simulink model "motor_velocity_2dof"  (R2014b)
settings: Solver=VariableStepAuto  StartTime=0.0  StopTime=simtime  RelTol=1e-3
values from neighbouring files (symbols this model uses):
  enable_karnop = 0    [discrete_velocity.m]    (also in ex1.m = 1; motor_parameters.mat = 1; pcontrol.m; pcontrol_position.m)
  enable_sin = 0    [discrete_velocity.m]    (also in ex1.m = 1; motor_parameters.mat; pcontrol.m = 1; pcontrol_position.m = 1)
  F_c = 1e-3    (= 0.001)    [ex1.m]    (also in motor_parameters.mat; position_ctrl.m; velocity_ctrl.m)
  J = J1+J2    (= 3.6e-05)    [ex1.m]    (also in lec_example.m = 0.1; position_ctrl.m = motor.J; velocity_ctrl.m)
  motor = motor_pars    [ex1.m]    (also in position_ctrl.m; velocity_ctrl.m)
  n = 5    [ex1.m]    (also in motor_parameters.mat; position_ctrl.m; velocity_ctrl.m)
  R = 1    [pcontrol.m]    (also in pcontrol_position.m; pdcontroller_position.m = [1 r0]; picontroller.m = [1 0]; picontroller_position.m = [1 r0])
  S = P    (= 8)    [pcontrol.m]    (also in pcontrol_position.m = 4; pdcontroller_position.m = [s1 s0]; picontroller.m = [P I]; picontroller_position.m = [s1 s0])
  sim_sin_amp = 200    [ex1.m]    (also in motor_parameters.mat = 1; pcontrol.m = 10; pcontrol_position.m = 10; pdcontroller_position.m = 10)
  sim_sin_freq = 10    [ex1.m]    (also in motor_parameters.mat = 1; pcontrol.m = 1; pcontrol_position.m = 1; pdcontroller_position.m = 1)
  sim_v = Vmax    (= 24)    [ex1.m]    (also in motor_parameters.mat; pcontrol.m = 1; pcontrol_position.m = 1; pdcontroller_position.m = 1)
  T = P    (= 8)    [pcontrol.m]    (also in pcontrol_position.m = 4; pdcontroller_position.m = S; picontroller.m = t0*[1 omega2]; picontroller_position.m = S)
libraries: simulink x2
settings Model: Creator=Gabriel  LastModifiedBy=gabras
settings DataIOCC: SaveFormat=Dataset
settings OptimizationCC: UseDivisionForNetSlopeComputation=off  SimCompilerOptimization=off
settings DebuggingCC: SolverPrmCheckMsg=none  FrameProcessingCompatibilityMsg=error  AllowSymbolicDim=off
settings HardwareCC: ProdBitPerPointer=64  ProdLargestAtomicFloat=Float  ProdIntDivRoundTo=Zero  ProdEndianess=LittleEndian  ProdWordSize=64  ProdHWDeviceType=Intel->x86-64 (Windows64)
settings RTWCC: RTWCompilerOptimization=off
settings GRTTargetCC: GeneratePreprocessorConditionals=Use local settings
settings ConfigComp: CovMetricSettings=dw  CovHtmlReporting=on  CovSaveCumulativeToWorkspaceVar=on  CovSaveSingleToWorkspaceVar=on  CovExternalEMLEnable=off

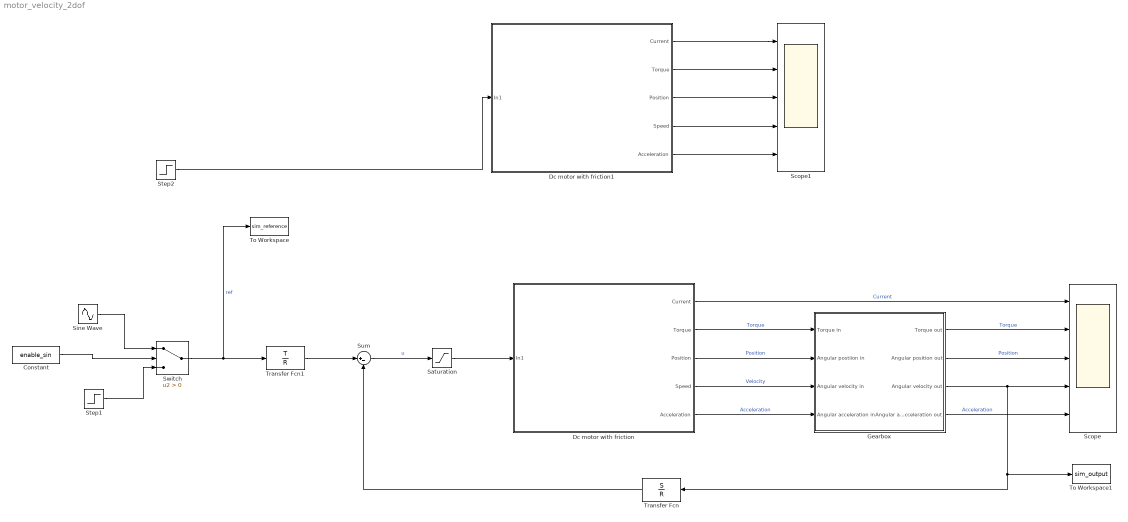
== system motor_velocity_2dof ==
  Constant : Constant  Value=enable_sin
  Dc motor with friction : Subsystem
      mask Display:
      | image('dcmotor.jpg')
      | port_label('input', 1, 'Voltage')
      | port_label('output', 1, 'Current')
      | port_label('output', 2, 'Torque')
      | port_label('output', 3, 'Position')
      | port_label('output', 4, 'Velocity')
      | port_label('output', 5, 'Acceleration')
  Dc motor with friction1 : Subsystem
      mask Display:
      | image('dcmotor.jpg')
      | port_label('input', 1, 'Voltage')
      | port_label('output', 1, 'Current')
      | port_label('output', 2, 'Torque')
      | port_label('output', 3, 'Position')
      | port_label('output', 4, 'Velocity')
      | port_label('output', 5, 'Acceleration')
  Gearbox : Subsystem
  Saturation : Saturate  UpperLimit=24  LowerLimit=-24
  Scope : Scope  NumInputPorts=5
      settings: YMin=-0.7198~-0.25085~-1.49914~-4.86523~-4731.79  YMax=1.13271~0.39475~13.4923~43.7871~7102.06
  Scope1 : Scope  NumInputPorts=5
      settings: YMin=-0.7198~-0.25085~-1.49914~-4.86523~-4731.79  YMax=1.13271~0.39475~13.4923~43.7871~7102.06
  Sine Wave : Sin  Amplitude=sim_sin_amp  Frequency=sim_sin_freq  SampleTime=0
  Step1 : Step  Time=0  After=sim_v  SampleTime=0
  Step2 : Step  Time=0  SampleTime=0
  Sum : Sum  Inputs=|+-
  Switch : Switch  Criteria=u2 > Threshold
  To Workspace : ToWorkspace  VariableName=sim_reference  SaveFormat=Timeseries  SampleTime=-1
  To Workspace1 : ToWorkspace  VariableName=sim_output  SaveFormat=Timeseries  SampleTime=-1
  Transfer Fcn : TransferFcn  Numerator=S  Denominator=R
  Transfer Fcn1 : TransferFcn  Numerator=T  Denominator=R
  wires:
  Step1/1 -> Switch/3
  Sine Wave/1 -> Switch/1
  Constant/1 -> Switch/2
  Switch/1 -> Transfer Fcn1/1, To Workspace/1  "ref"
  Dc motor with friction/4(Speed) -> Gearbox/3(Angular velocity in)  "Velocity"
  Dc motor with friction/2(Torque) -> Gearbox/1(Torque in)  "Torque"
  Dc motor with friction/1(Current) -> Scope/1  "Current"
  Dc motor with friction/5(Acceleration) -> Gearbox/4(Angular acceleration in)  "Acceleration"
  Dc motor with friction/3(Position) -> Gearbox/2(Angular postiion in)  "Position"
  Gearbox/1(Torque out) -> Scope/2  "Torque"
  Gearbox/2(Angular position out) -> Scope/3  "Position"
  Gearbox/3(Angular velocity out) -> To Workspace1/1, Transfer Fcn/1, Scope/4
  Gearbox/4(Angular acceleration out) -> Scope/5  "Acceleration"
  Transfer Fcn/1 -> Sum/2
  Transfer Fcn1/1 -> Sum/1
  Sum/1 -> Saturation/1  "u"
  Dc motor with friction1/1(Current) -> Scope1/1
  Dc motor with friction1/2(Torque) -> Scope1/2
  Dc motor with friction1/3(Position) -> Scope1/3
  Dc motor with friction1/4(Speed) -> Scope1/4
  Dc motor with friction1/5(Acceleration) -> Scope1/5
  Step2/1 -> Dc motor with friction1/1(In1)
  Saturation/1 -> Dc motor with friction/1(In1)

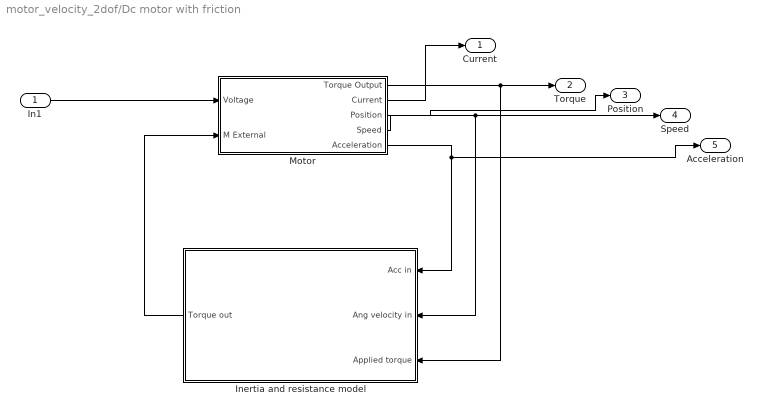
== system motor_velocity_2dof/Dc motor with friction ==
  In1 : Inport
  "Inertia and resistance model " : Subsystem
  Motor : Subsystem
  Current : Outport
  Torque : Outport  Port=2
  Position : Outport  Port=3
  Speed : Outport  Port=4
  Acceleration : Outport  Port=5
  wires:
  Motor/4(Speed) -> Speed/1, "Inertia and resistance model "/2(Ang velocity in)
  Motor/3(Position) -> Position/1
  Motor/2(Current) -> Current/1
  "Inertia and resistance model "/1(Torque out) -> Motor/2("M External ")
  Motor/1(Torque Output) -> Torque/1, "Inertia and resistance model "/3(Applied torque)
  In1/1 -> Motor/1(Voltage)
  Motor/5(Acceleration) -> "Inertia and resistance model "/1(Acc in), Acceleration/1

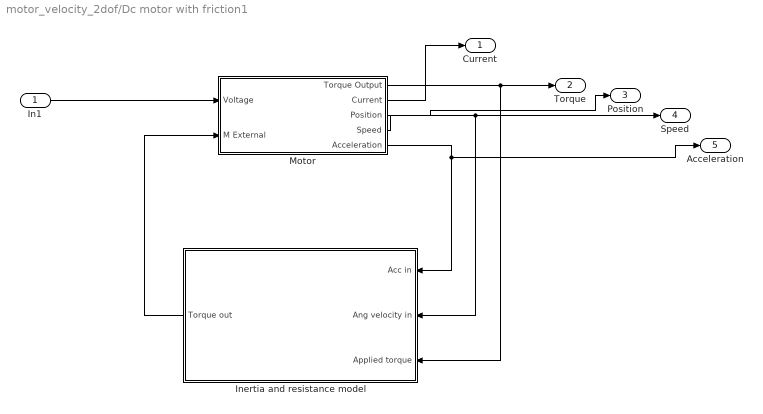
== system motor_velocity_2dof/Dc motor with friction1 ==
  In1 : Inport
  "Inertia and resistance model " : Subsystem
  Motor : Subsystem
  Current : Outport
  Torque : Outport  Port=2
  Position : Outport  Port=3
  Speed : Outport  Port=4
  Acceleration : Outport  Port=5
  wires:
  Motor/5(Acceleration) -> Acceleration/1, "Inertia and resistance model "/1(Acc in)
  In1/1 -> Motor/1(Voltage)
  Motor/1(Torque Output) -> "Inertia and resistance model "/3(Applied torque), Torque/1
  "Inertia and resistance model "/1(Torque out) -> Motor/2("M External ")
  Motor/2(Current) -> Current/1
  Motor/3(Position) -> Position/1
  Motor/4(Speed) -> "Inertia and resistance model "/2(Ang velocity in), Speed/1

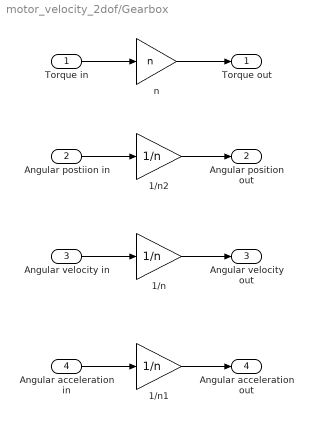
== system motor_velocity_2dof/Gearbox ==
  Torque in : Inport
  Angular postiion in : Inport  Port=2
  Angular velocity in : Inport  Port=3
  Angular acceleration in : Inport  Port=4
  1/n : Gain  Gain=1/n
  1/n1 : Gain  Gain=1/n
  1/n2 : Gain  Gain=1/n
  n : Gain  Gain=n
  Torque out : Outport
  Angular position out : Outport  Port=2
  Angular velocity out : Outport  Port=3
  Angular acceleration out : Outport  Port=4
  wires:
  1/n/1 -> Angular velocity out/1
  Angular velocity in/1 -> 1/n/1
  n/1 -> Torque out/1
  Torque in/1 -> n/1
  1/n1/1 -> Angular acceleration out/1
  Angular acceleration in/1 -> 1/n1/1
  1/n2/1 -> Angular position out/1
  Angular postiion in/1 -> 1/n2/1

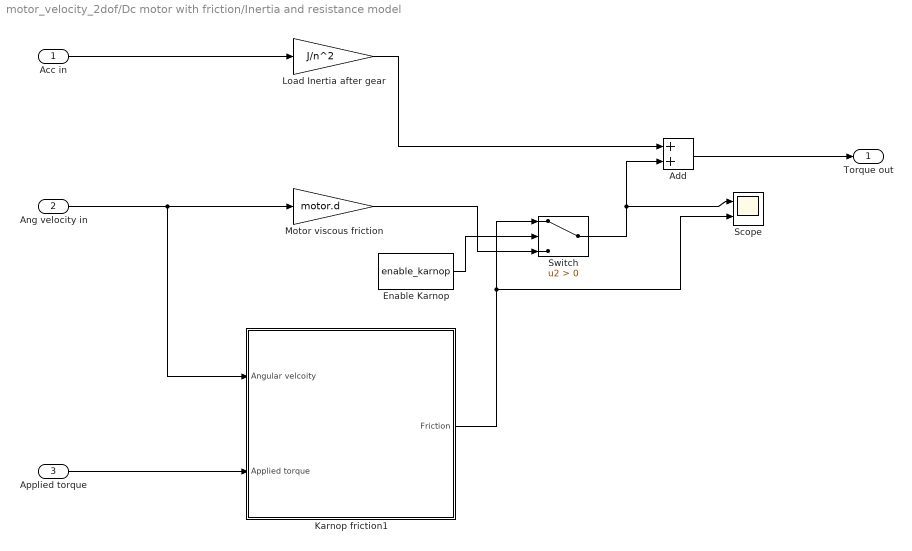
== system motor_velocity_2dof/Dc motor with friction/Inertia and resistance model  ==
  Acc in : Inport
  Ang velocity in : Inport  Port=2
  Applied torque : Inport  Port=3
  Add : Sum
  Enable Karnop : Constant  Value=enable_karnop
  Karnop friction1 : Subsystem
  Load Inertia after gear : Gain  Gain=J/n^2
  Motor viscous friction : Gain  Gain=motor.d
  Scope : Scope  NumInputPorts=2
      settings: YMin=-0.00177~-0.00177  YMax=0.00177~0.00177
  Switch : Switch  Criteria=u2 > Threshold
  Torque out : Outport
  wires:
  Acc in/1 -> Load Inertia after gear/1
  Add/1 -> Torque out/1
  Load Inertia after gear/1 -> Add/1
  Ang velocity in/1 -> Karnop friction1/1(Angular velcoity), Motor viscous friction/1
  Motor viscous friction/1 -> Switch/3
  Karnop friction1/1(Friction) -> Switch/1, Scope/2
  Switch/1 -> Add/2, Scope/1
  Enable Karnop/1 -> Switch/2
  Applied torque/1 -> Karnop friction1/2("Applied torque ")

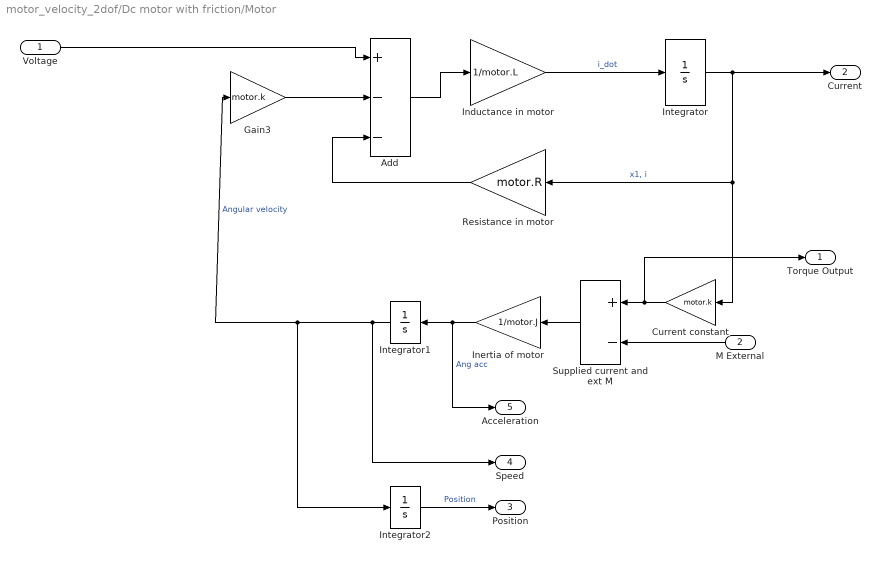
== system motor_velocity_2dof/Dc motor with friction/Motor ==
  Voltage : Inport
  "M External " : Inport  Port=2
  Add : Sum  Inputs=+--
  Current constant : Gain  Gain=motor.k
  Gain3 : Gain  Gain=motor.k
  Inductance in motor : Gain  Gain=1/motor.L
  Inertia of motor : Gain  Gain=1/motor.J
  Integrator : Integrator
  Integrator1 : Integrator
  Integrator2 : Integrator
  Resistance in motor : Gain  Gain=motor.R
  "Supplied current and ext M " : Sum  Inputs=+-
  Torque Output : Outport
  Current : Outport  Port=2
  Position : Outport  Port=3
  Speed : Outport  Port=4
  Acceleration : Outport  Port=5
  wires:
  Voltage/1 -> Add/1
  Add/1 -> Inductance in motor/1
  Inductance in motor/1 -> Integrator/1  "i_dot"
  Integrator/1 -> Current constant/1, Resistance in motor/1, Current/1  "x1, i"
  Resistance in motor/1 -> Add/3
  Gain3/1 -> Add/2
  Integrator1/1 -> Speed/1, Integrator2/1, Gain3/1  "Angular velocity"
  "Supplied current and ext M "/1 -> Inertia of motor/1
  Inertia of motor/1 -> Acceleration/1, Integrator1/1  "Ang acc"
  Current constant/1 -> Torque Output/1, "Supplied current and ext M "/1
  "M External "/1 -> "Supplied current and ext M "/2
  Integrator2/1 -> Position/1  "Position"

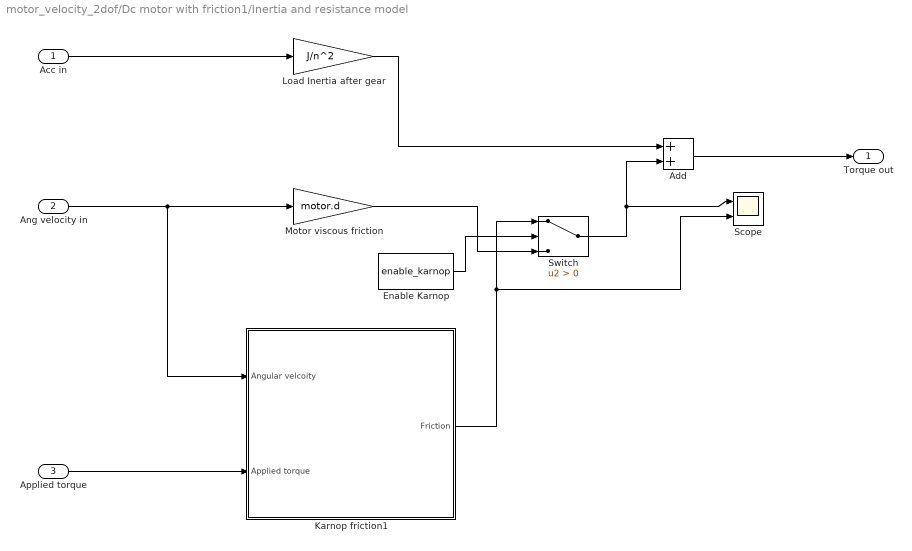
== system motor_velocity_2dof/Dc motor with friction1/Inertia and resistance model  ==
  Acc in : Inport
  Ang velocity in : Inport  Port=2
  Applied torque : Inport  Port=3
  Add : Sum
  Enable Karnop : Constant  Value=enable_karnop
  Karnop friction1 : Subsystem
  Load Inertia after gear : Gain  Gain=J/n^2
  Motor viscous friction : Gain  Gain=motor.d
  Scope : Scope  NumInputPorts=2
      settings: YMin=-0.00177~-0.00177  YMax=0.00177~0.00177
  Switch : Switch  Criteria=u2 > Threshold
  Torque out : Outport
  wires:
  Applied torque/1 -> Karnop friction1/2("Applied torque ")
  Enable Karnop/1 -> Switch/2
  Switch/1 -> Scope/1, Add/2
  Karnop friction1/1(Friction) -> Scope/2, Switch/1
  Motor viscous friction/1 -> Switch/3
  Ang velocity in/1 -> Motor viscous friction/1, Karnop friction1/1(Angular velcoity)
  Load Inertia after gear/1 -> Add/1
  Add/1 -> Torque out/1
  Acc in/1 -> Load Inertia after gear/1

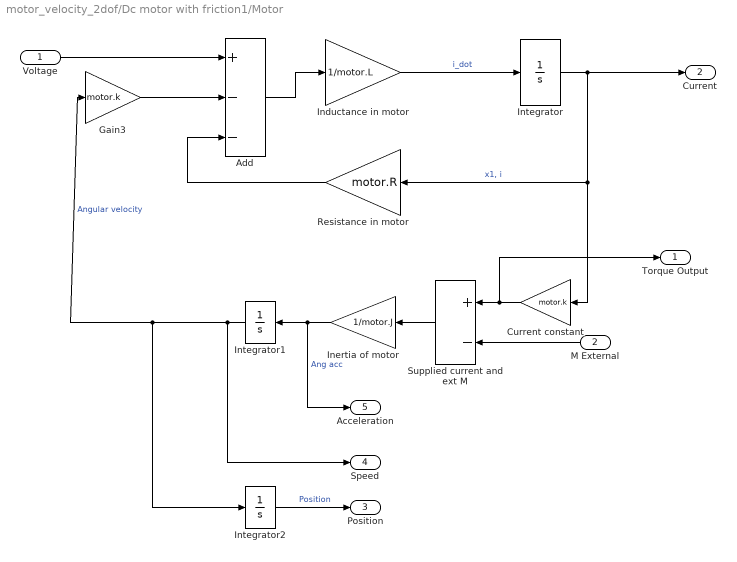
== system motor_velocity_2dof/Dc motor with friction1/Motor ==
  Voltage : Inport
  "M External " : Inport  Port=2
  Add : Sum  Inputs=+--
  Current constant : Gain  Gain=motor.k
  Gain3 : Gain  Gain=motor.k
  Inductance in motor : Gain  Gain=1/motor.L
  Inertia of motor : Gain  Gain=1/motor.J
  Integrator : Integrator
  Integrator1 : Integrator
  Integrator2 : Integrator
  Resistance in motor : Gain  Gain=motor.R
  "Supplied current and ext M " : Sum  Inputs=+-
  Torque Output : Outport
  Current : Outport  Port=2
  Position : Outport  Port=3
  Speed : Outport  Port=4
  Acceleration : Outport  Port=5
  wires:
  Integrator2/1 -> Position/1  "Position"
  "M External "/1 -> "Supplied current and ext M "/2
  Current constant/1 -> "Supplied current and ext M "/1, Torque Output/1
  Inertia of motor/1 -> Integrator1/1, Acceleration/1  "Ang acc"
  "Supplied current and ext M "/1 -> Inertia of motor/1
  Integrator1/1 -> Gain3/1, Integrator2/1, Speed/1  "Angular velocity"
  Gain3/1 -> Add/2
  Resistance in motor/1 -> Add/3
  Integrator/1 -> Current/1, Resistance in motor/1, Current constant/1  "x1, i"
  Inductance in motor/1 -> Integrator/1  "i_dot"
  Add/1 -> Inductance in motor/1
  Voltage/1 -> Add/1

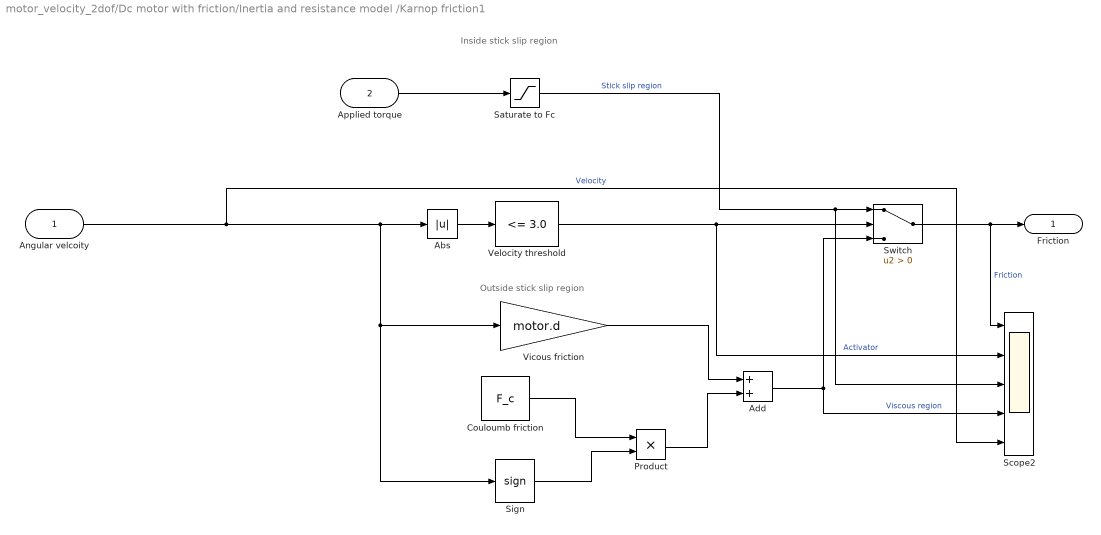
== system motor_velocity_2dof/Dc motor with friction/Inertia and resistance model /Karnop friction1 ==
  note: Inside stick slip region
  note: Outside stick slip region
  Angular velcoity : Inport
  "Applied torque " : Inport  Port=2
  Abs : Abs
  Add : Sum
  Couloumb friction : Constant  Value=F_c
  Product : Product
  Saturate to Fc : Saturate  UpperLimit=F_c  LowerLimit=-F_c
  Scope2 : Scope  NumInputPorts=5
      settings: ShowLegends=on  YMin=-0.00177~-0.125~0.0009~-0.00177~-138.1533~-0.12501~-0.12501~-0.12501  YMax=0.00177~1.125~0.0011~0.00177~138.10681~0.12501~0.12501~0.12501  SaveName=ScopeData3
  Sign : Signum
  Switch : Switch  Criteria=u2 > Threshold
  "Velocity threshold " : simulink/Logic and Bit Operations/Compare To Constant  relop=<=  const=3.0  OutDataTypeStr=boolean
  Vicous friction : Gain  Gain=motor.d
  Friction : Outport
  wires:
  Saturate to Fc/1 -> Scope2/3, Switch/1  "Stick slip region"
  Switch/1 -> Scope2/1, Friction/1  "Friction"
  Angular velcoity/1 -> Scope2/5, Abs/1, Vicous friction/1, Sign/1  "Velocity"
  "Velocity threshold "/1 -> Scope2/2, Switch/2  "Activator"
  Abs/1 -> "Velocity threshold "/1
  Product/1 -> Add/2
  Vicous friction/1 -> Add/1
  Couloumb friction/1 -> Product/1
  Sign/1 -> Product/2
  "Applied torque "/1 -> Saturate to Fc/1
  Add/1 -> Switch/3, Scope2/4  "Viscous region"

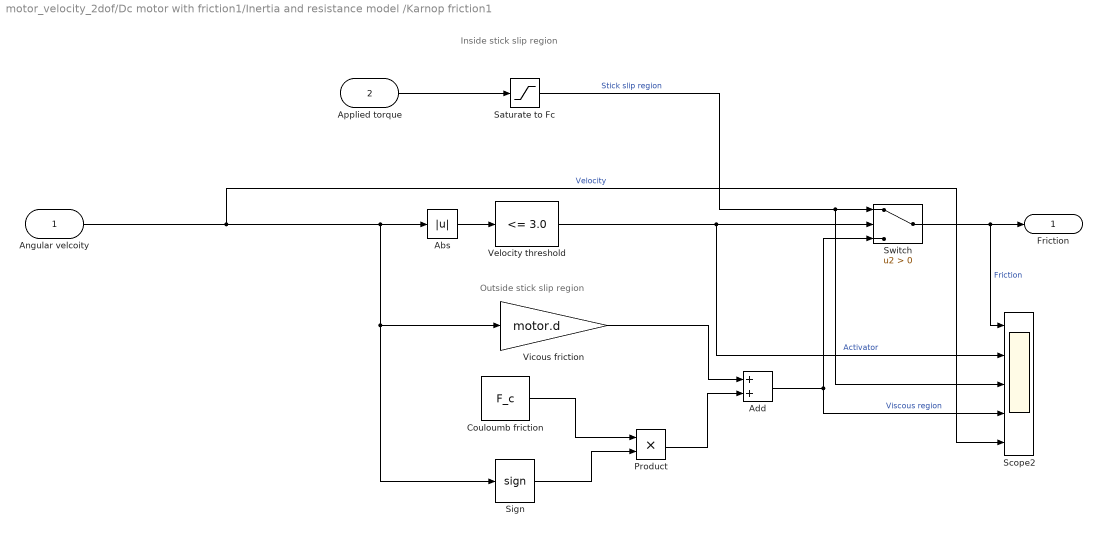
== system motor_velocity_2dof/Dc motor with friction1/Inertia and resistance model /Karnop friction1 ==
  note: Outside stick slip region
  note: Inside stick slip region
  Angular velcoity : Inport
  "Applied torque " : Inport  Port=2
  Abs : Abs
  Add : Sum
  Couloumb friction : Constant  Value=F_c
  Product : Product
  Saturate to Fc : Saturate  UpperLimit=F_c  LowerLimit=-F_c
  Scope2 : Scope  NumInputPorts=5
      settings: ShowLegends=on  YMin=-0.00177~-0.125~0.0009~-0.00177~-138.1533~-0.12501~-0.12501~-0.12501  YMax=0.00177~1.125~0.0011~0.00177~138.10681~0.12501~0.12501~0.12501  SaveName=ScopeData3
  Sign : Signum
  Switch : Switch  Criteria=u2 > Threshold
  "Velocity threshold " : simulink/Logic and Bit Operations/Compare To Constant  relop=<=  const=3.0  OutDataTypeStr=boolean
  Vicous friction : Gain  Gain=motor.d
  Friction : Outport
  wires:
  Add/1 -> Scope2/4, Switch/3  "Viscous region"
  "Applied torque "/1 -> Saturate to Fc/1
  Sign/1 -> Product/2
  Couloumb friction/1 -> Product/1
  Vicous friction/1 -> Add/1
  Product/1 -> Add/2
  Abs/1 -> "Velocity threshold "/1
  "Velocity threshold "/1 -> Switch/2, Scope2/2  "Activator"
  Angular velcoity/1 -> Sign/1, Vicous friction/1, Abs/1, Scope2/5  "Velocity"
  Switch/1 -> Friction/1, Scope2/1  "Friction"
  Saturate to Fc/1 -> Switch/1, Scope2/3  "Stick slip region"
